simulink model "trial"  (R2020b)
settings: Solver=VariableStepAuto  StartTime=0.0  StopTime=5e4  RelTol=1e-3
libraries: cstblocks x1
settings Model: OrderedModelArguments=off  Creator=Jamesh  LastModifiedBy=HP

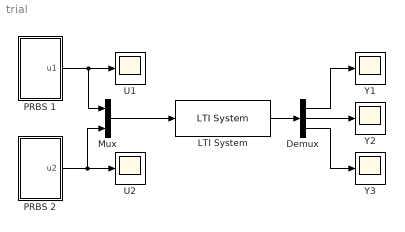
== system trial ==
  Demux : Demux  Outputs=3
  LTI System : cstblocks/LTI System  sys=sys  IC=[]
  Mux : Mux  Inputs=2
  PRBS 1 : Subsystem
  PRBS 2 : Subsystem
  U1 : Scope
  U2 : Scope
  Y1 : Scope
  Y2 : Scope
  Y3 : Scope
  wires:
  Mux/1 -> LTI System/1
  LTI System/1 -> Demux/1
  Demux/1 -> Y1/1
  Demux/2 -> Y2/1
  Demux/3 -> Y3/1
  PRBS 1/1(u1) -> U1/1, Mux/1
  PRBS 2/1(u2) -> U2/1, Mux/2

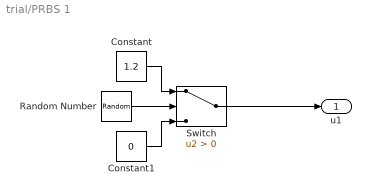
== system trial/PRBS 1 ==
  Constant : Constant  Value=1.2
  Constant1 : Constant  Value=0
  Random Number : RandomNumber  Seed=1  SampleTime=0.25
  Switch : Switch  Criteria=u2 > Threshold
  u1 : Outport
  wires:
  Switch/1 -> u1/1
  Random Number/1 -> Switch/2
  Constant1/1 -> Switch/3
  Constant/1 -> Switch/1

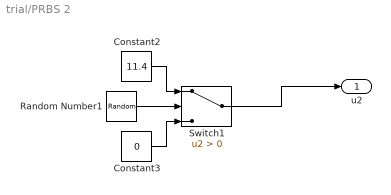
== system trial/PRBS 2 ==
  Constant2 : Constant  Value=11.4
  Constant3 : Constant  Value=0
  Random Number1 : RandomNumber  Seed=2  SampleTime=0.25
  Switch1 : Switch  Criteria=u2 > Threshold
  u2 : Outport
  wires:
  Random Number1/1 -> Switch1/2
  Switch1/1 -> u2/1
  Constant3/1 -> Switch1/3
  Constant2/1 -> Switch1/1
